simulink model "active_suspension_kalman_sim"  (R2017b)
settings: Solver=ode45  StartTime=0.0  StopTime=20.0  MaxStep=0.001  RelTol=1e-3  EnableMultiTasking=on
values from neighbouring files (symbols this model uses):
  A = [[0 1 0 0 0];[-(cw+cs)/mw -ds/mw cs/mw ds/mw -1/mw];[0 0 0 1 0];[cs/mc ds/mc -cs/mc -ds/mc 1/mc];[0 0 0 0 -1/tau]]    [active_suspension_kalman_design.m]
  B1 = [B H]    [active_suspension_kalman_design.m]
  B2 = [B L]    [active_suspension_kalman_design.m]
  C = [-1 0 1 0 0]    [active_suspension_kalman_design.m]
  C1 = eye(5)    [active_suspension_kalman_design.m]
  D1 = zeros(5,2)    [active_suspension_kalman_design.m]
settings Model: Creator=JonasMac  LastModifiedBy=jofr
settings DataIOCC: LimitDataPoints=on  SaveFormat=Array
settings OptimizationCC: LifeSpan=inf
settings DebuggingCC: UnderspecifiedInitializationDetection=Classic  MergeDetectMultiDrivingBlocksExec=none  SolverPrmCheckMsg=warning  SFUnexpectedBacktrackingDiag=warning  SFNoUnconditionalDefaultTransitionDiag=warning  SFExecutionAtInitializationDiag=none
settings HardwareCC: ProdBitPerPointer=32  ProdBitPerSizeT=32  ProdBitPerPtrDiffT=32  ProdLargestAtomicFloat=None  ProdIntDivRoundTo=Undefined  ProdEndianess=Unspecified  ProdWordSize=32  ProdHWDeviceType=32-bit Generic
settings ModelReferenceCC: PropagateSignalLabelsOutOfModel=off
settings CodeAppCC: StateflowObjectComments=on
settings GRTTargetCC: TargetLangStandard=C89/C90 (ANSI)  GeneratePreprocessorConditionals=Disable all
settings ConfigComp: CovMetricSettings=dw  CovHtmlReporting=on  CovSaveCumulativeToWorkspaceVar=on  CovSaveSingleToWorkspaceVar=on  CovExternalEMLEnable=off

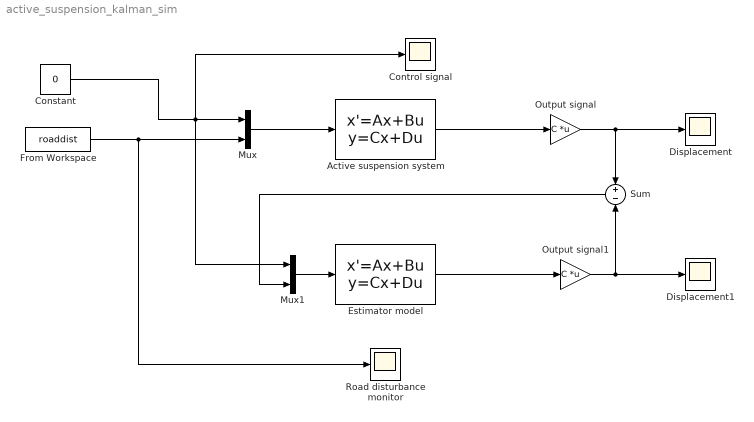
== system active_suspension_kalman_sim ==
  Active suspension system : StateSpace  A=A  B=B1  C=C1  D=D1  InitialCondition=0
  Constant : Constant  Value=0
  Control signal : Scope
  Displacement : Scope
  Displacement1 : Scope
  Estimator model : StateSpace  A=A  B=B2  C=C1  D=D1  InitialCondition=0
  From Workspace : FromWorkspace  VariableName=roaddist  SampleTime=0
  Mux : Mux  Inputs=2
  Mux1 : Mux  Inputs=2
  Output signal : Gain  Gain=C  Multiplication=Matrix(K*u)
  Output signal1 : Gain  Gain=C  Multiplication=Matrix(K*u)
  Road disturbance monitor : Scope
  Sum : Sum  Inputs=+|-
  wires:
  Output signal/1 -> Displacement/1, Sum/1
  Active suspension system/1 -> Output signal/1
  Mux/1 -> Active suspension system/1
  From Workspace/1 -> Mux/2, Road disturbance monitor/1
  Output signal1/1 -> Sum/2, Displacement1/1
  Mux1/1 -> Estimator model/1
  Estimator model/1 -> Output signal1/1
  Sum/1 -> Mux1/2
  Constant/1 -> Control signal/1, Mux1/1, Mux/1
